simulink library "aerolibbdyn"  (Simulink 5.0)
libraries: fixpt_lib_4 x3, aerolibschedule x2, simulink x2, aerolibutil x2
settings Model: Creator=sgage  LastModifiedBy=sgage  ExtModeAutoUpdateStatusClock=off  TargetHWChar=2  TargetHWWordLengths=8,16,32,32

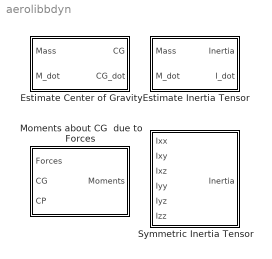
== system aerolibbdyn ==
  Estimate Center of Gravity : Subsystem  mask(Estimate Center of Gravity){fmass=2, emass=1, fcg=[1 1 1]', ecg=[0.5 0.5 0.5]'}
      mask prompts: fmass "Full mass:"; emass "Empty mass:"; fcg "Full center of gravity:"; ecg "Empty center of gravity:"
      mask help: Calculate the center of gravity location. Linear interpolation is used to determine center of gravity as a function of mass.
      mask init:
      | cg(:,:,1)=ecg;
      | cg(:,:,2)=fcg;
      | 
      | [x y xp yp]=aeroimage('cg');
      mask Help: web(asbhelp);
      mask Display:
      | port_label('input',1,'mass','texmode','on');
      | port_label('input',2,'dm/dt','texmode','on');
      | port_label('output',1,'CG','texmode','on');
      | port_label('output',2,'dCG/dt','texmode','on');
      | patch(xp,yp);
      | patch(x,y,[1 1 1]);
  Estimate Inertia Tensor : Subsystem  mask(Estimate Inertia Tensor){fmass=2, emass=1, fI=eye(3), eI=eye(3)/2}
      mask prompts: fmass "Full mass:"; emass "Empty mass:"; fI "Full inertia matrix:"; eI "Empty inertia matrix:"
      mask help: Calculate the inertia tensor. Linear interpolation is used to determine inertia tensor as a function of mass.
      mask init:
      | I(:,:,1)=eI;
      | I(:,:,2)=fI;
      | [xp yp xp2 yp2]=aeroimage('inertia');
      mask Help: web(asbhelp);
      mask Display:
      | port_label('input',1,'mass','texmode','on');
      | port_label('input',2,'dm/dt','texmode','on');
      | port_label('output',1,'I','texmode','on');
      | port_label('output',2,'dI/dt','texmode','on');
      | patch(xp,yp);
      | patch(xp2,yp2);
  Moments about CG  due to Forces : Subsystem  mask(Moments About CG Due To Forces){}
      mask help: Compute moments about center of gravity due to forces which are applied at point CP not the center of gravity.
      mask init:
      | [xpw ypw xp yp x y]=aeroimage('momcg');
      mask Help: web(asbhelp);
      mask Display:
      | port_label('input',1,'F','texmode','on');
      | port_label('input',2,'CG','texmode','on');
      | port_label('input',3,'CP','texmode','on');
      | port_label('output',1,'M','texmode','on');
      | patch(xp,yp);
      | patch(xpw,ypw,[1 1 1]);
      | plot(x,y);
  Symmetric Inertia Tensor : Subsystem  mask(Symmetric Inertia Tensor){}
      mask help: Create an inertia tensor from moments and products of inertia. Each input corresponds to an element of the tensor.
      mask init:
      | [xp yp xp2 yp2]=aeroimage('inertia');
      mask Help: web(asbhelp);
      mask Display:
      | port_label('input',1,'I_{xx}','texmode','on');
      | port_label('input',2,'I_{xy}','texmode','on');
      | port_label('input',3,'I_{xz}','texmode','on');
      | port_label('input',4,'I_{yy}','texmode','on');
      | port_label('input',5,'I_{yz}','texmode','on');
      | port_label('input',6,'I_{zz}','texmode','on');
      | port_label('output',1,'I','texmode','on');
      | patch(xp,yp);
      | patch(xp2,yp2);

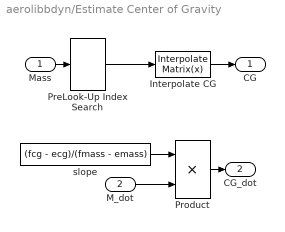
== system aerolibbdyn/Estimate Center of Gravity ==
  Mass : Inport
  M_dot : Inport  Port=2
  Interpolate CG : aerolibschedule/Interpolate Matrix(x)  matrix=cg
  PreLook-Up Index Search : simulink/Look-Up Tables/PreLook-Up Index Search  bpData=[emass fmass]  searchMode=Binary Search  cacheBpFlag=off  outputFlag=off  extrapMode=Clip to Range  rangeErrorMode=None
  Product : Product  SaturateOnIntegerOverflow=on
  slope : Constant  Value=(fcg - ecg)/(fmass - emass)
  CG : Outport
  CG_dot : Outport  Port=2
  wires:
  slope/1 -> Product/1
  M_dot/1 -> Product/2
  Product/1 -> CG_dot/1
  Mass/1 -> PreLook-Up Index Search/1
  Interpolate CG/1 -> CG/1
  PreLook-Up Index Search/1 -> Interpolate CG/1

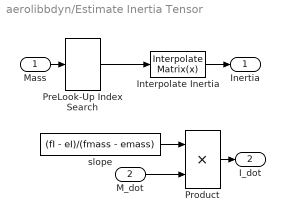
== system aerolibbdyn/Estimate Inertia Tensor ==
  Mass : Inport
  M_dot : Inport  Port=2
  Interpolate Inertia : aerolibschedule/Interpolate Matrix(x)  matrix=I
  PreLook-Up Index Search : simulink/Look-Up Tables/PreLook-Up Index Search  bpData=[emass fmass]  searchMode=Binary Search  cacheBpFlag=off  outputFlag=off  extrapMode=Clip to Range  rangeErrorMode=None
  Product : Product  SaturateOnIntegerOverflow=on
  slope : Constant  Value=(fI - eI)/(fmass - emass)
  Inertia : Outport
  I_dot : Outport  Port=2
  wires:
  slope/1 -> Product/1
  M_dot/1 -> Product/2
  Product/1 -> I_dot/1
  PreLook-Up Index Search/1 -> Interpolate Inertia/1
  Interpolate Inertia/1 -> Inertia/1
  Mass/1 -> PreLook-Up Index Search/1

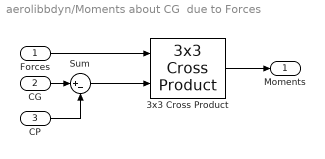
== system aerolibbdyn/Moments about CG  due to Forces ==
  Forces : Inport
  CG : Inport  Port=2
  CP : Inport  Port=3
  3x3 Cross Product : aerolibutil/3x3 Cross Product
  Sum : Sum  Inputs=|+-  SaturateOnIntegerOverflow=on
  Moments : Outport
  wires:
  CG/1 -> Sum/1
  CP/1 -> Sum/2
  3x3 Cross Product/1 -> Moments/1
  Forces/1 -> 3x3 Cross Product/1
  Sum/1 -> 3x3 Cross Product/2

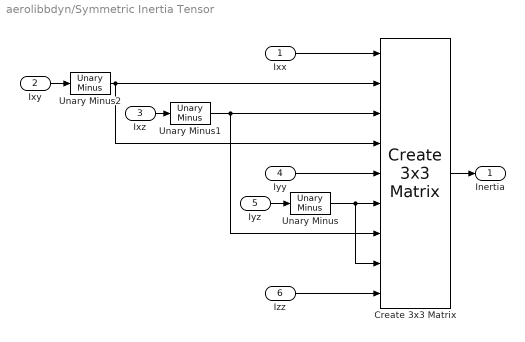
== system aerolibbdyn/Symmetric Inertia Tensor ==
  Ixx : Inport
  Ixy : Inport  Port=2
  Ixz : Inport  Port=3
  Iyy : Inport  Port=4
  Iyz : Inport  Port=5
  Izz : Inport  Port=6
  Create 3x3 Matrix : aerolibutil/Create 3x3 Matrix
  Unary Minus : fixpt_lib_4/Math/Unary Minus  DoSatur=off
  Unary Minus1 : fixpt_lib_4/Math/Unary Minus  DoSatur=off
  Unary Minus2 : fixpt_lib_4/Math/Unary Minus  DoSatur=off
  Inertia : Outport
  wires:
  Unary Minus2/1 -> Create 3x3 Matrix/2, Create 3x3 Matrix/4
  Unary Minus1/1 -> Create 3x3 Matrix/3, Create 3x3 Matrix/7
  Unary Minus/1 -> Create 3x3 Matrix/6, Create 3x3 Matrix/8
  Izz/1 -> Create 3x3 Matrix/9
  Iyz/1 -> Unary Minus/1
  Create 3x3 Matrix/1 -> Inertia/1
  Iyy/1 -> Create 3x3 Matrix/5
  Ixz/1 -> Unary Minus1/1
  Ixy/1 -> Unary Minus2/1
  Ixx/1 -> Create 3x3 Matrix/1
